simulink model "mainECU"  (R2015b)
settings: Solver=FixedStepDiscrete  StartTime=0.0  StopTime=Inf  FixedStep=0.001  RelTol=1e-3
PostLoadFcn:
  | , if any(exist('dsrtsu_mdlpostloadfcn', 'file') == [2, 3, 6]), try dsrtsu_mdlpostloadfcn('Execute', bdroot); catch fprintf('Error in PostLoadFcn (dsrtsu_mdlpostloadfcn) for model "%s":\n %s\n', bdroot, lasterr); end, end,
undefined symbols (not defined in the file or in its folder): STARTUP
libraries: dspswit3 x5, rtican x5, simulink x2
(part 1 of 2)
settings Model: DSRTSU_INTERNAL_RTI_VER=460  DSRTSU_INTERNAL_RTI_TYPE=rti1401  RTICANMMDATA=struct('GeneralSetupData',struct('modelroot','e:\working\ds1401\demos\model\ds1401\model','generalsettings',struct('filesettings',struct('destfolder',struct('Name','RTICANMM_FILES','Check',1),'buildfolder',struct('Name','.','Check',1),'AbsDestfolder',struct('Name','e:\working\ds1401\demos\model\ds1401\model\RTICANMM_FILES'),'AbsBuildfolder',struct('Name','e:\working\ds1401\demos\model\ds1401\model'))),'options',struct('addpaths',1,'rmpaths',1,'addtrcexclusion',logical(1),'cannavigator',struct('checkmonitoring',0),'show_usrtrc',0,'use_usrtrc',0),'advanced',struct('options',[1 1 1 1 1 1 1 1 1 1 1 1 1 1 1 1 1 1 1 1 1 1 1 1 1 1 1 1 1 1 1 1 1 1 1 1 1 1 1 1 1 1 1 1 1 1 1 1 1 1 1 1 1 1 1 1 1 1 1 1 1 1 1 1 1 1 1 1 1 1 1 1 1 1 1 1 1 1 1 1 1 1 1 1 1 1 1 1 1 1 1 1 1 1 1 1 1 1 1 1]),'MPSetup',{{}},'modelname','demo1401_throttle_control_1513','block','demo1401_throttle_control_1513'))  DSRTSU_INTERNAL_RTIFLEXRAYCONFIG=70  DSRTSU_INTERNAL_RTIFPGA=50  ExtModeTrigMode=oneshot  ExtModeArmWhenConnect=off  ExtModeAutoUpdateStatusClock=off  Creator=dSPACE GmbH  LastModifiedBy=luis
settings SolverCC: AutoInsertRateTranBlk=on
settings DataIOCC: SaveFormat=Array  SignalLoggingSaveFormat=ModelDataLogs
settings OptimizationCC: BlockReduction=off  ConditionallyExecuteInputs=off  OptimizeBlockIOStorage=off  BufferReuse=off  GlobalBufferReuse=off  ExpressionFolding=off  ExpressionDepthLimit=2147483647  LocalBlockOutputs=off  InitFltsAndDblsToZero=on
settings DebuggingCC: SaveWithParameterizedLinksMsg=none  UnderspecifiedInitializationDetection=Classic  MergeDetectMultiDrivingBlocksExec=none  SignalResolutionControl=TryResolveAllWithWarning  SolverPrmCheckMsg=warning  MultiTaskDSMMsg=warning  MultiTaskCondExecSysMsg=none  MultiTaskRateTransMsg=warning  TasksWithSamePriorityMsg=none  FcnCallInpInsideContextMsg=UseLocalSettings  StateNameClashWarn=warning
settings HardwareCC: ProdBitPerPointer=32  ProdLargestAtomicFloat=None  ProdEndianess=BigEndian  ProdWordSize=32  ProdHWDeviceType=Generic->Custom  TargetIntDivRoundTo=Zero  TargetEndianess=BigEndian  TargetHWDeviceType=Generic->Custom
settings RTWCC: SystemTargetFile=rti1401.tlc  MakeCommand=make_rti  TemplateMakefile=rti1401.tmf  Description=dSPACE DS1401 Hardware Platform  RTWVerbose=off
settings STFCustomTargetCC: ParMdlRefBuildCompliant=on  ConcurrentExecutionCompliant=off  GeneratePreprocessorConditionals=Use local settings  CPPClassGenCompliant=off  SystemTargetFile=rti1401.tlc
settings GRTTargetCC: CompOptLevelCompliant=off  ConcurrentExecutionCompliant=off  CombineOutputUpdateFcns=off  MatFileLogging=off  CPPClassGenCompliant=off  GRTInterface=on  UseToolchainInfoCompliant=off  ExtModeMexFile=noextcomm
settings ConfigComp: CovModelRefEnable=Off

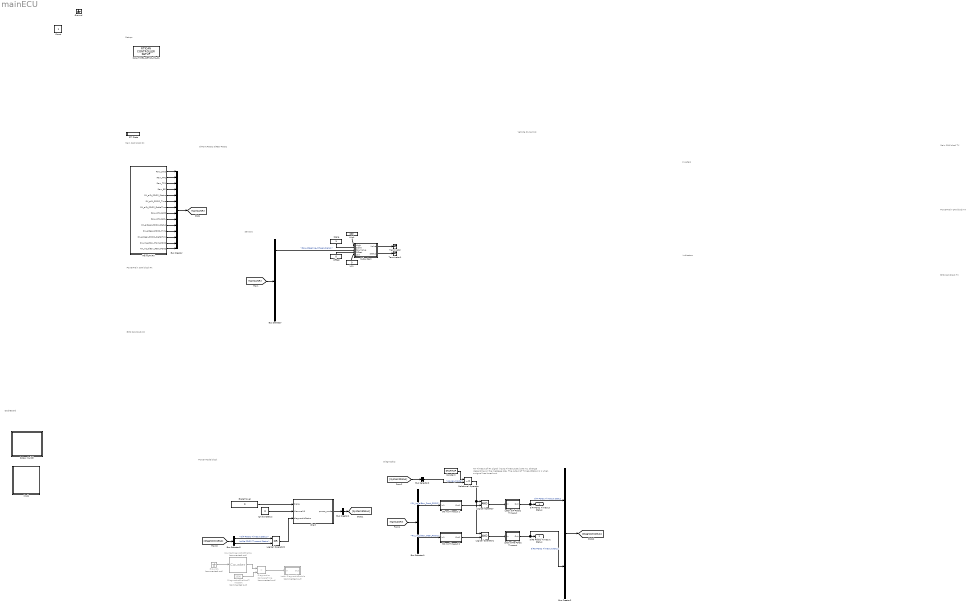
== system mainECU ==
  note: DashBoard
  note: Diagnostics
  note: RX Timeout of RX signal inputs
      | Timeout set is 50 ms. Change depending on the message rate.
      | The output of TimeoutStatus is 1 when a signal has timed out.
  note: aiFront PDO2
      | aiRear PDO2
  note: Sensors
  note: Power Mode block
  note: Main
      | CAN block
      | RX
  note: Setups
  note: PowerTrain
      | CAN block
      | RX
  note: BMS
      | CAN block
      | RX
  note: Vehicle Dynamics
  note: Indicators
  note: Inverters
  note: Main
      | CAN block
      | TX
  note: PowerTrain
      | CAN block
      | TX
  note: BMS
      | CAN block
      | TX
  50 ms Timeout 1 : Subsystem
  50 ms Timeout 2 : Subsystem
  BrakeTravel : Constant  Value=0
  Bus Creator : BusCreator  Inputs=14
  Bus Creator1 : BusCreator  Inputs=1
  Bus Creator2 : BusCreator  Inputs=2
  Bus Selector : BusSelector  OutputSignals=Raw_Steering_Wheel_Signal,Raw_Throttle_Pedal_2,Raw_Throttle_Pedal_1,Raw_Brake_Signal
  Bus Selector1 : BusSelector  OutputSignals=RX_Int_aiBox_Front_PDO2,RX_Int_aiBox_Rear_PDO2
  Bus Selector2 : BusSelector  OutputSignals=power_mode
  Bus Selector3 : BusSelector  OutputSignals=aiFr PDO2 Timeout Status,aiRe PDO2 Timeout Status
  CAN_TYPE1_SETUP_M1_C1 : rtican/RTICAN CONTROLLER SETUP   Reserved1=[]  Reserved2=[]  Reserved3=[]  Reserved4=[]  AcceptanceMask=[]  ArbitrationField=[]  Parameters=[]  SFcnRTICANSettings=[]  MS_Struct=[]  BoardTypeNo=[]  BoardNo=[]  ChannelNo=[]  DialogFcn=[]  UnitName=[]  Revision=[]  UnitValues=[]  DSProperties=struct('RTI',struct('Version',uint32(12),'BlockType',struct('isSLSource',uint8(0),'isSLSink',uint8(0),'isHWSource',uint8(0),'isHWSink',uint8(0),'isSetup',uint8(1),'isInline',uint8(1),'isNonInline',uint8(0),'isInterrupt',uint8(0),'isChannelwise',uint8(0)),'IOBoardType','RTICAN','UnitType','NON_MESSAGE','Identifier','MASTER','DialogType','ML','BlockSet','RTICAN','SlaveProcessor','CAN'))  RTIBlockInterface=struct('InputPortsWidth',int32(0),'InputPortsActive',0,'OutputPortsWidth',int32(0),'OutputPortsActive',0,'DialogFcn','rtican_master_setup_gui','BlockDisplay',{{['CAN CONTROLLER\n SETUP'],'center'}},'IconTransparency','on','InitLevel',3,'IWork',{{{'',uint32(2)}}},'BlockName',struct('Token',{{'CAN_TYPE','_SETUP_M','_C'}},'BlockParam',{{'BoardTypeNo','BoardNo','ChannelNo'}}),'ParameterTunableNames',{{}})  RTIBlockParameters="struct('BoardTypeNo',{{1,'OFF',[]}},'BoardNo',{{1,'ON',[1 16]}},'ChannelNo',{{1,'ON',[1 2]}},'AcceptanceMask',{{0,'OFF',[]}},'ArbitrationField',{{0,'OFF',[]}},'Parameters',{{struct('Config',struct('Baudrate',500,'SampleMode',1,'UsedParamSet',1,'validSettings',1,'isBTRvalues',0,'Advanced',struct('Baudrate',{500,500,500},'Frequency',{24000000,36000000,64000000},'Settings',{struct('SMPL',0,'BRP',0,'NBT',24,'TSEG1',15,'TSEG2',6,'SJW',3,'SP',70),struct('SMPL',0,'BRP',1,'NBT',18,'TSEG1',14,'TSEG2',1,'SJW',1,'SP',88),struct('SMPL',0,'BRP',3,'NBT',16,'TSEG1',12,'TSEG2',1,'SJW',1,'SP',87)},'BTR0',{192,65,67},'BTR1',{111,30,28})),'configType',1,'Options',struct('DataFileSelected',1,'DataFileName',{{'database\\main_0_2.dbc'}},'DataFileDate',{{['07-ene.-2017 20:06:27']}},'InterfaceFcn','rtican_dbc_file_parser','InterfaceFcnFileName','','LabelConfigType','volatile','AcceptanceMaskSelected',0,'MsgDataType','AllwaysDouble','NumType','hex','MaskType','STD','AcceptanceMask',0,'ArbitrationField',0,'UseMultipleMessageAccess',0),'RxReceiveStdOptions',struct('RxServiceStdEnabled',0,'RxServiceStdMsgIdent',1000,'RxServiceStdIdentNumType',1,'RxServiceStdIdentMask',0,'RxServiceStdMaskNumType',1,'RxServiceStdQueueSize',64),'RxReceiveXtdOptions',struct('RxServiceXtdEnabled',0,'RxServiceXtdMsgIdent',1001,'RxServiceXtdIdentNumType',1,'RxServiceXtdIdentMask',0,'RxServiceXtdMaskNumType',1,'RxServiceXtdQueueSize',64),'PartialNetworkingOptions',struct('switchedon',0,'format',1,'idmask',['    XXXXX XXXXXXXX XXXXXXXX XXXXXXXX'],'idcode','0','idfilter','0','datamaskused',0,'datalength',1,'datamask','0x0000000000000000','partialnetworkenable',0),'general',struct('Termination_common',1,'Termination_C252',1,'BusConfigurationRegister',0,'Transceiver','ISO11898','isFromLib',0)),'OFF',[]}},'CCPParameters',{{struct('CRO',struct('Format','STD','NumFormat','hex','Id',1639),'DTO',struct('Format','STD','NumFormat','hex','Id',2017),'StationAdr',struct('NumFormat','hex','Value',57),'StationId',struct('Value',['dSPACE CCP Service']),'Enabled',0),'OFF',[]}},'XCPParameters',{{struct('MASTER',struct('Format','STD','NumFormat','hex','Id',256),'SLAVE',struct('Format','STD','NumFormat','hex','Id',510),'Enabled',0,'PIDTransmissionEnabled',0),'OFF',[]}},'GroupId',{{struct('Group',{{'RTICAN'}},'No',1,'Behavior',{{'EVER'}},'BlockType',{{'SOURCE'}},'NameChangeFlag',1),'OFF',[]}},'SFcnRTICANSettings',{{struct('Baudrate',500,'configType',1,'AdvancedConfig',struct('Frequency',{},'BTR0',{},'BTR1',{}),'UsedParamSet',1,'STDMaskSelected','no','XTDMaskSelected','no','BoardType','DS1','BoardNo',1,'ControllerNo',1,'Transceiver','ISO11898','BusConfigRegister',0,'TerminationRes',120,'UseMultipleMessageAccess','no','STDRXSrvcUsed','no','STDRXSrvcMsgId',1000,'STDRXSrvcMsgMask',0,'STDRXSrvcQueueSize',64,'XTDRXSrvcUsed','no','XTDRXSrvcMsgId',1001,'XTDRXSrvcQueueSize',64,'XTDRXSrvcMsgMask',0,'PN_IsPNTransciever',0,'PN_IsPNEnabled',0,'PN_MsgFormat',1,'PN_idcode',0,'PN_idmask',2047,'PN_datamaskused',0,'PN_datalength',0,'PN_datamask',['0xFF, 0xFF, 0xFF, 0xFF, 0xFF, 0xFF, 0xFF, 0xFF']),'OFF',[]}},'SFcnRTICCPSettings',{{struct('CRO',struct('Format','STD','NumFormat','hex','Id',1639),'DTO',struct('Format','STD','NumFormat','hex','Id',2017),'StationAdr',struct('NumFormat','hex','Value',57),'StationId',struct('Value',['dSPACE CCP Service']),'Enabled',0),'OFF',[]}},'SFcnRTIXCPSettings',{{struct('MASTER',struct('Format','STD','NumFormat','hex','Id',256),'SLAVE',struct('Format','STD','NumFormat','hex','Id',510),'Enabled',0,'PIDTransmissionEnabled',0),'OFF',[]}},'TLCFileName',{{'rtican_master_setup','OFF',[]}})"  RTISFcnParameters=struct('SFcnRTICANSettings','struct','SFcnRTICCPSettings','struct','SFcnRTIXCPSettings','struct','AcceptanceMask','int32','ArbitrationField','int32','TLCFileName','char')  RTIBlockParaDefault="struct('BoardTypeNo',4302,'BoardNo',1,'ChannelNo',1,'AcceptanceMask',0,'ArbitrationField',0,'Parameters',struct('Config',struct('Baudrate',500,'SampleMode',1,'UsedParamSet',1,'validSettings',1,'isBTRvalues',0,'Advanced',struct('Frequency',16000000,'BTR0',64,'BTR1',28,'Settings',struct('SMPL',0,'BRP',0,'NBT',16,'TSEG1',12,'TSEG2',1,'SJW',1,'SP',87))),'configType',1,'Options',struct('DataFileSelected',0,'DataFileName',{{['<no datafile support>']}},'DataFileDate',{{''}},'InterfaceFcn','rtican_dbc_file_parser','InterfaceFcnFileName','','LabelConfigType','volatile','AcceptanceMaskSelected',0,'MsgDataType','AllwaysDouble','NumType','hex','MaskType','STD','AcceptanceMask',0,'ArbitrationField',0,'UseMultipleMessageAccess',0),'RxReceiveStdOptions',struct('RxServiceStdEnabled',0,'RxServiceStdMsgIdent',1000,'RxServiceStdIdentNumType',1,'RxServiceStdIdentMask',0,'RxServiceStdMaskNumType',1,'RxServiceStdQueueSize',64),'RxReceiveXtdOptions',struct('RxServiceXtdEnabled',0,'RxServiceXtdMsgIdent',1001,'RxServiceXtdIdentNumType',1,'RxServiceXtdIdentMask',0,'RxServiceXtdMaskNumType',1,'RxServiceXtdQueueSize',64),'PartialNetworkingOptions',struct('switchedon',0,'format',1,'idmask',['    XXXXX XXXXXXXX XXXXXXXX XXXXXXXX'],'idcode','0','idfilter','0','datamaskused',0,'datalength',1,'datamask','0x0000000000000000','partialnetworkenable',0),'general',struct('Termination_common',1,'Termination_C252',1,'BusConfigurationRegister',0,'Transceiver','ISO11898','isFromLib',1)),'CCPParameters',struct('CRO',struct('Format','STD','NumFormat','hex','Id',1639),'DTO',struct('Format','STD','NumFormat','hex','Id',2017),'StationAdr',struct('NumFormat','hex','Value',57),'StationId',struct('Value',['dSPACE CCP Service']),'Enabled',0),'XCPParameters',struct('MASTER',struct('Format','STD','NumFormat','hex','Id',256),'SLAVE',struct('Format','STD','NumFormat','hex','Id',510),'Enabled',0,'PIDTransmissionEnabled',0),'GroupId',struct('Group',{{'RTICAN'}},'No',1,'Behavior',{{'EVER'}},'BlockType',{{'SOURCE'}},'NameChangeFlag',1),'SFcnRTICANSettings',struct('Baudrate',500,'configType',1,'AdvandedConfig',struct('Frequency',16000000,'BTR0','0x40','BTR1','0x1C'),'UsedParamSet',1,'STDMaskSelected','no','XTDMaskSelected','no','BoardType','DS4302','BoardNo',1,'ControllerNo',1,'Transceiver','ISO11898','BusConfigRegister',0,'TerminationRes',120,'UseMultipleMessageAccess','no','STDRXSrvcUsed','no','STDRXSrvcMsgId',1000,'STDRXSrvcMsgMask',0,'STDRXSrvcQueueSize',64,'XTDRXSrvcUsed','no','XTDRXSrvcMsgId',1001,'XTDRXSrvcQueueSize',64,'XTDRXSrvcMsgMask',0),'SFcnRTICCPSettings',struct('CRO',struct('Format','STD','NumFormat','hex','Id',1639),'DTO',struct('Format','STD','NumFormat','hex','Id',2017),'StationAdr',struct('NumFormat','hex','Value',57),'StationId',struct('Value',['dSPACE CCP Service']),'Enabled',0),'SFcnRTIXCPSettings',struct('MASTER',struct('Format','STD','NumFormat','hex','Id',256),'SLAVE',struct('Format','STD','NumFormat','hex','Id',510),'Enabled',0,'PIDTransmissionEnabled',0),'TLCFileName','rtican_master_setup')"
      settings: AttributesFormatString=Group Id: RTICAN1\n
  Chart : Stateflow chart  TreatAsAtomicUnit=on
  Constant : Constant  Value=STARTUP
  CounterDiagnosticsEnable : dspswit3/Counter  Commented=on  Direction=Up  CountEvent=Free running  CounterSize=User defined  MaxCount=20000  InitialCount=0  Output=Count  HitValue=32  ResetInput=on  SamplesPerFrame=1  Ts=-1  CntDtype=double  HitDtype=Logical
  Diagnostics CompareTime : RelationalOperator  Commented=on  Operator=>  OutDataTypeStr=boolean
  DiagnosticsEnabledTimeStart : Constant  Commented=on  Value=2000
  Ground1 : Ground  Commented=on
  High : Constant  Value=100
  IgnitionStatus : Constant  Value=0
  Knob : Subsystem  DialogController=hmiCreateDDGDialog  IsWebBlock=on  mask(MWDashboardBlock){webBlockId=318b6eff-2907-45e0-b318-c643b2e3d79c, webBlockType=continuousknob, ShowInLibBrowser=on, ShowInitialText=on, HMISrcModelName=mainECU}
      mask prompts: webBlockId "WebBlock Id"; webBlockType "WebBlock Type"; HMISrcModelName "Source Model"
      mask Help: helpview([docroot '/mapfiles/simulink.map'], 'hmi_knob')
      mask Display:
      | if strcmp(get_param(bdroot(gcb),'BlockDiagramType'), 'library')
      |     image([(matlabroot) '/toolbox/simulink/hmi/icons/ContinuousKnob.png']);
      | end
  Latch DiagnosticEnable : Subsystem  Commented=on
  Latch aiFr PDO2 Timeout : Subsystem
  Latch aiRe PDO2 Timeout : Subsystem
  Logical Operator : Logic  AllPortsSameDT=off  OutDataTypeStr=boolean
  Logical Operator1 : Logic  AllPortsSameDT=off  OutDataTypeStr=boolean
  Logical Operator2 : Logic  Operator=OR  AllPortsSameDT=off  OutDataTypeStr=boolean
  Low : Constant  Value=0
  MainCAN RX : Subsystem
  Offset : Constant  Value=0
  RTI Data : Subsystem  Tag=struct('RTIDataServer',struct('RTIDataServerVs','2','RTIModelDescription','struct(''main'',''mainECU'',''sub'','''',''isMp'',0)'))  LoadFcn="if exist('rtidc'), try,  rtidc('DataHostBlockClbLoad', gcbh); catch, disp(['Warning: ''LoadFcn'' for RTI Data block failed: ' lasterr]); end, end,"  mask(RTI_DATA_HOST){}
      mask help:
      | RTI Data Block.
      | This block is used by RTI to store internal model-dependent data.
      | Please keep this block on the root level of the model. Deleting this block will result in data loss.
      |
      | NEVER DELETE OR COPY THIS BLOCK!
      settings: CopyFcn="if exist('rtidc'), try,  rtidc('DataHostBlockClbCopy', gcbh); catch, disp(['Warning: ''CopyFcn'' for RTI Data block failed: ' lasterr]); end, end,"  DeleteFcn="if exist('rtidc'), try,  rtidc('DataHostBlockClbDelete', gcbh); catch, disp(['Warning: ''DeleteFcn'' for RTI Data block failed: ' lasterr]); end, end,"  ModelCloseFcn="if exist('rtidc'), try,  rtidc('DataHostBlockClbModelClose', gcbh); catch, disp(['Warning: ''ModelCloseFcn'' for RTI Data block failed: ' lasterr]); end, end,"  PreSaveFcn="if exist('rtidc'), try,  rtidc('DataHostBlockClbPreSave', gcbh); catch, disp(['Warning: ''PreSaveFcn'' for RTI Data block failed: ' lasterr]); end, end,"  PostSaveFcn="if exist('rtidc'), try,  rtidc('DataHostBlockClbPostSave', gcbh); catch, disp(['Warning: ''PostSaveFcn'' for RTI Data block failed: ' lasterr]); end, end,"  NameChangeFcn="if exist('rtidc'), try,  rtidc('DataHostBlockClbNameChange', gcbh); catch, disp(['Warning: ''NameChangeFcn'' for RTI Data block failed: ' lasterr]); end, end,"
      mask Help:
      | RTI Data Block.
      | This block is used by RTI to store internal model-dependent data.
      | Please keep this block on the root level of the model. Deleting this block will result in data loss.
      | 
      | NEVER DELETE OR COPY THIS BLOCK!
      mask Display:
      | text(0.5, 0.5, 'RTI Data', 'HorizontalAlignment', 'center');
      | plot([1 0]);
  Relational Operator : RelationalOperator  Operator=~=  OutDataTypeStr=boolean
  Rotary Switch : Subsystem  DialogController=hmiCreateDDGDialog  IsWebBlock=on  mask(MWDashboardBlock){webBlockId=394b7d7a-f303-4d15-a706-6c693a0bf5c3, webBlockType=discreteknob, ShowInLibBrowser=on, ShowInitialText=on, HMISrcModelName=mainECU}
      mask prompts: webBlockId "WebBlock Id"; webBlockType "WebBlock Type"; HMISrcModelName "Source Model"
      mask Help: helpview([docroot '/mapfiles/simulink.map'], 'hmi_rotary_switch')
      mask Display:
      | model = bdroot(gcb);
      | if strcmp(get_param(model,'BlockDiagramType'), 'library')
      |     image([(matlabroot) '/toolbox/simulink/hmi/icons/DiscreteKnob.png']);
      | end
  Scale : Constant
  Subsystem : Subsystem
  Terminator : Terminator
  Terminator1 : Terminator
  aiFr PDO2 Timeout Status : Outport
  aiRe PDO2 Timeout Status : Outport  Port=2
  Const : Constant  IOType=siggen
  Ground : Ground  IOType=siggen
  tag scope: MainCANRX=global
  wires:
  MainCAN RX/6(RX_aiFr_PDO2_Time) -> Bus Creator/6
  MainCAN RX/1(Raw_SWS) -> Bus Creator/1
  MainCAN RX/2(Raw_TP2) -> Bus Creator/2
  MainCAN RX/3(Raw_TP1) -> Bus Creator/3
  MainCAN RX/4("Raw_BS ") -> Bus Creator/4
  MainCAN RX/5(RX_aiFr_PDO2_Status) -> Bus Creator/5
  MainCAN RX/7(RX_aiFr_PDO2_DeltaTime) -> Bus Creator/7
  MainCAN RX/8(Raw_WSuspRR) -> Bus Creator/8
  MainCAN RX/9(Raw_WSuspRL) -> Bus Creator/9
  MainCAN RX/10(RX_aiRear_PDO2_Status) -> Bus Creator/10
  MainCAN RX/11(RX_aiRear_PDO2_Time) -> Bus Creator/11
  MainCAN RX/12(RX_aiRear_PDO2_DeltaTime) -> Bus Creator/12
  [MainCANRX] -> Bus Selector/1
  Bus Creator/1 -> [MainCANRX]
  [MainCANRX] -> Bus Selector1/1
  MainCAN RX/13(RX_Int_aiBox_Front_PDO2) -> Bus Creator/13
  MainCAN RX/14(RX_Int_aiBox_Rear_PDO2) -> Bus Creator/14
  Bus Selector1/2 -> 50 ms Timeout 2/1(In1)  "<RX_Int_aiBox_Rear_PDO2>"
  Bus Selector1/1 -> 50 ms Timeout 1/1(In1)  "<RX_Int_aiBox_Front_PDO2>"
  50 ms Timeout 1/1(Out1) -> Logical Operator/2
  [SystemStatus] -> Bus Selector2/1
  Bus Creator1/1 -> [SystemStatus]
  50 ms Timeout 2/1(Out1) -> Logical Operator1/2
  Ground1/1 -> CounterDiagnosticsEnable/1
  DiagnosticsEnabledTimeStart/1 -> Diagnostics CompareTime/2
  CounterDiagnosticsEnable/1 -> Diagnostics CompareTime/1
  Logical Operator1/1 -> Latch aiRe PDO2 Timeout/1(In)
  Logical Operator/1 -> Latch aiFr PDO2 Timeout/1(In)
  Latch aiFr PDO2 Timeout/1(Out) -> Bus Creator2/1, aiFr PDO2 Timeout Status/1  "aiFr PDO2 Timeout Status"
  Latch aiRe PDO2 Timeout/1(Out) -> Bus Creator2/2, aiRe PDO2 Timeout Status/1  "aiRe PDO2 Timeout Status"
  Diagnostics CompareTime/1 -> Latch DiagnosticEnable/1(In)
  High/1 -> Subsystem/1(High)
  Scale/1 -> Subsystem/2(Scale)
  Bus Selector/1 -> Subsystem/3(RawValue)  "<Raw_Steering_Wheel_Signal>"
  Offset/1 -> Subsystem/4(Offset)
  Low/1 -> Subsystem/5(Low)
  Subsystem/1(Value) -> Terminator/1
  Subsystem/2(Status) -> Terminator1/1
  Chart/1(power_mode) -> Bus Creator1/1
  IgnitionStatus/1 -> Chart/2(klemme15)
  BrakeTravel/1 -> Chart/1(brake)
  Bus Creator2/1 -> [DiagnosticsBus]
  [DiagnosticsBus] -> Bus Selector3/1
  Bus Selector3/1 -> Logical Operator2/1  "<aiFr PDO2 Timeout Status>"
  Bus Selector3/2 -> Logical Operator2/2  "<aiRe PDO2 Timeout Status>"
  Logical Operator2/1 -> Chart/3(diagnosticStatus)
  Relational Operator/1 -> Logical Operator1/1, Logical Operator/1
  Bus Selector2/1 -> Relational Operator/2  "<power_mode>"
  Constant/1 -> Relational Operator/1

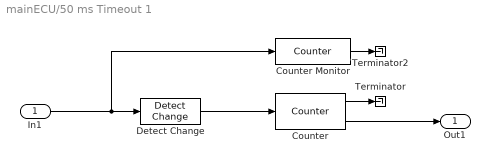
== system mainECU/50 ms Timeout 1 ==
  In1 : Inport
  Counter : dspswit3/Counter  Direction=Up  CountEvent=Free running  CounterSize=User defined  MaxCount=65535  InitialCount=0  Output=Count and Hit  HitValue=55  ResetInput=on  SamplesPerFrame=1  Ts=-1  CntDtype=double  HitDtype=Boolean
  Counter Monitor : dspswit3/Counter  Direction=Up  CountEvent=Either edge  CounterSize=User defined  MaxCount=100000  InitialCount=0  Output=Count  HitValue=32  ResetInput=off  SamplesPerFrame=1  Ts=1  CntDtype=double  HitDtype=Logical
  Detect Change : simulink/Logic and Bit Operations/Detect Change  vinit=0  InputProcessing=Inherited  OutDataTypeStr=uint8
  Terminator : Terminator
  Terminator2 : Terminator
  Out1 : Outport
  wires:
  Counter Monitor/1 -> Terminator2/1
  Counter/2 -> Out1/1
  Counter/1 -> Terminator/1
  In1/1 -> Counter Monitor/1, Detect Change/1
  Detect Change/1 -> Counter/1

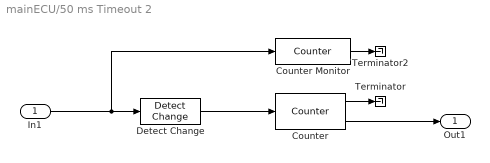
== system mainECU/50 ms Timeout 2 ==
  In1 : Inport
  Counter : dspswit3/Counter  Direction=Up  CountEvent=Free running  CounterSize=User defined  MaxCount=65535  InitialCount=0  Output=Count and Hit  HitValue=55  ResetInput=on  SamplesPerFrame=1  Ts=-1  CntDtype=double  HitDtype=Boolean
  Counter Monitor : dspswit3/Counter  Direction=Up  CountEvent=Either edge  CounterSize=User defined  MaxCount=100000  InitialCount=0  Output=Count  HitValue=32  ResetInput=off  SamplesPerFrame=1  Ts=1  CntDtype=double  HitDtype=Logical
  Detect Change : simulink/Logic and Bit Operations/Detect Change  vinit=0  InputProcessing=Inherited  OutDataTypeStr=uint8
  Terminator : Terminator
  Terminator2 : Terminator
  Out1 : Outport
  wires:
  Counter Monitor/1 -> Terminator2/1
  Counter/2 -> Out1/1
  Counter/1 -> Terminator/1
  In1/1 -> Counter Monitor/1, Detect Change/1
  Detect Change/1 -> Counter/1

== system mainECU/Knob ==

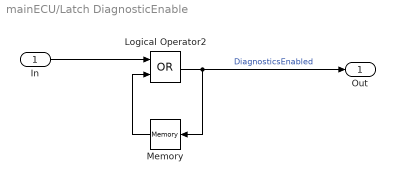
== system mainECU/Latch DiagnosticEnable ==
  In : Inport  OutDataTypeStr=boolean
  Logical Operator2 : Logic  Operator=OR  OutDataTypeStr=boolean
  Memory : Memory  X0=false
  Out : Outport
  wires:
  Memory/1 -> Logical Operator2/2
  Logical Operator2/1 -> Out/1, Memory/1  "DiagnosticsEnabled"
  In/1 -> Logical Operator2/1

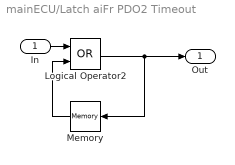
== system mainECU/Latch aiFr PDO2 Timeout ==
  In : Inport
  Logical Operator2 : Logic  Operator=OR  AllPortsSameDT=off  OutDataTypeStr=boolean
  Memory : Memory
  Out : Outport
  wires:
  Memory/1 -> Logical Operator2/2
  In/1 -> Logical Operator2/1
  Logical Operator2/1 -> Memory/1, Out/1

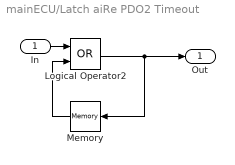
== system mainECU/Latch aiRe PDO2 Timeout ==
  In : Inport
  Logical Operator2 : Logic  Operator=OR  AllPortsSameDT=off  OutDataTypeStr=boolean
  Memory : Memory
  Out : Outport
  wires:
  Memory/1 -> Logical Operator2/2
  In/1 -> Logical Operator2/1
  Logical Operator2/1 -> Memory/1, Out/1

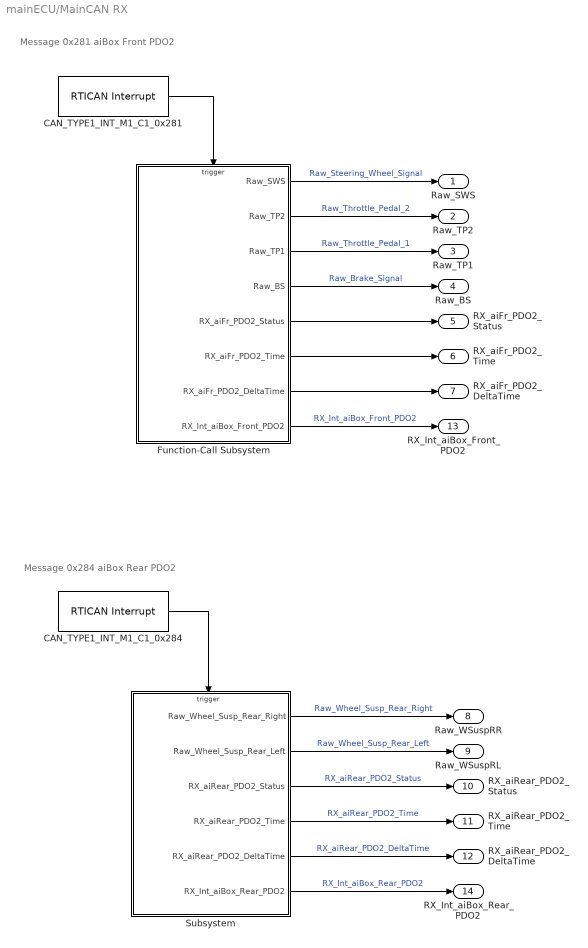
== system mainECU/MainCAN RX ==
  note: Message 0x284 aiBox Rear PDO2
  note: Message 0x281 aiBox Front PDO2
  CAN_TYPE1_INT_M1_C1_0x281 : rtican/RTICAN Interrupt  Reserved1=[]  Reserved2=[]  Reserved3=[]  Reserved4=[]  BoardTypeNo=[]  BoardNo=[]  ChannelNo=[]  Parameters=[]  InterruptName=[]  BoardIntNo=[]  Sfcn_Int_Struct=[]  BoardType=[]  SintNo=[]  Int_Struct=[]  DialogFcn=[]  UnitName=[]  Revision=[]  UnitValues=[]  DSProperties=struct('RTI',struct('Version',uint32(4),'BlockType',struct('isSLSource',uint8(1),'isSLSink',uint8(0),'isHWSource',uint8(1),'isHWSink',uint8(0),'isSetup',uint8(0),'isInline',uint8(1),'isNonInline',uint8(0),'isInterrupt',uint8(1),'isChannelwise',uint8(0)),'IOBoardType','RTICAN','UnitType','HWINT','Identifier','CANINT','DialogType','ML','BlockSet','RTICAN','RelationId',struct('TH',struct('BlockId','HWINT')),'SlaveProcessor','CAN'))  RTIBlockInterface=struct('OutputPortsWidth',int32(1),'FunctionCall',uint32(0),'OutputPortsActive',1,'DialogFcn','rtican_interrupt_gui','BlockDisplay',{{['CAN RX Interrupt'],'center'}},'IconTransparency','off','ParameterTunableNames',{{}},'InitLevel',3,'BlockName',struct('Token',{{'CAN_TYPE','_INT_M','_C'}},'BlockParam',{{'BoardTypeNo','BoardNo','ChannelNo'}}),'Options',{{'SS_OPTION_FORCE_NONINLINED_FCNCALL','SS_OPTION_ASYNCHRONOUS_INTERRUPT'}})  RTIBlockParameters=struct('BoardTypeNo',{{1,'OFF',[]}},'BoardNo',{{1,'ON',[1 16]}},'ChannelNo',{{1,'ON',[1 2]}},'Parameters',{{struct('general',struct('Type','RX','NumFormat','hex','MsgIdFormat','STD','MsgId',641,'isFromLib',0)),'OFF',[]}},'GroupId',{{struct('Group','RTICAN','No',1,'Behavior','NAMECHANGE','BlockType','SINK','NameChangeFlag',0),'OFF',[]}},'SFcnRTICANInterrupt',{{0,'OFF',[]}},'ThSrcSgnName',{{['CAN_TYPE1_M1_C1 RX Interrupt'],'OFF',[]}},'ThBlk',{{['struct(''blkh'',[''mainECU/MainCAN RX/CAN_TYPE1_INT_M1_C1_0x281''],''srcId'',''CAN1'',''srcSgnId'',''CAN1'',''intervalTmrBlockId'',[],''srcSgnName'',[''CAN_TYPE1_M1_C1 RX Interrupt''],''srcCpuId'','''',''isSrcCpu'',1,''isTargetCpu'',1,''srcOnMasterCpu'',1,''boardType'',''CAN'',''boardTypeNo'',''1'',''boardNo'',0,''intNo'',0,''subIntNo'',-1,''period'',0,''entryPoint'',''rti_CAN1'',''blockName'',''CAN_TYPE1_INT_M1_C1_0x281'',''taskNameDisplayExt'','''',''taskType'',''HWINT'',''groupId'',''CANINT1B1'',''hookFcn'',''NULL'',''isTimerTaskSrc'',0,''service'','''',''mpBlkId'','''',''taskPriorityPreConfig'',''none'',''taskPriority'',-1,''taskSortWeighting'',[],''taskSchedulingPolicy'',''FCFS'',''taskOvrPreConfig'',''none'',''taskOvrStrategy'',1,''taskOvrQueueSize'',1,''taskVisibility'',''on'',''taskGroupId'','''',''taskGroupDisplayOrder'',[],''serviceDynamicGen'',0,''disableCodeGen'',0,''boardBase'',''0'',''noBoardBase'','''')'],'OFF',[]}},'PHSBoardBaseId',{{'DS4302','OFF',[]}},'TLCFileName',{{'rtican_interrupt','OFF',[]}})  RTISFcnParameters=struct('SFcnRTICANInterrupt','struct','ThBlk','struct','PHSBoardBaseId','char','TLCFileName','char')  RTIBlockParaDefault=struct('BoardTypeNo',4302,'BoardNo',1,'ChannelNo',1,'Parameters',struct('general',struct('Type','RX','NumFormat','dec','MsgIdFormat','STD','MsgId',100,'isFromLib',1)),'GroupId',struct('Group',{{'RTICAN'}},'No',1,'Behavior',{{'NAMECHANGE'}},'BlockType',{{'SINK'}},'NameChangeFlag',0),'SFcnRTICANInterrupt',0,'ThSrcSgnName',['DS4302CAN_B1_C1 RX Interrupt'],'ThBlk',['struct(''srcSgnId'', '''')'],'PHSBoardBaseId','DS4302','TLCFileName','rtican_interrupt')
      settings: AttributesFormatString=Group Id: RTICAN1\n
  CAN_TYPE1_INT_M1_C1_0x284 : rtican/RTICAN Interrupt  Reserved1=[]  Reserved2=[]  Reserved3=[]  Reserved4=[]  BoardTypeNo=[]  BoardNo=[]  ChannelNo=[]  Parameters=[]  InterruptName=[]  BoardIntNo=[]  Sfcn_Int_Struct=[]  BoardType=[]  SintNo=[]  Int_Struct=[]  DialogFcn=[]  UnitName=[]  Revision=[]  UnitValues=[]  DSProperties=struct('RTI',struct('Version',uint32(4),'BlockType',struct('isSLSource',uint8(1),'isSLSink',uint8(0),'isHWSource',uint8(1),'isHWSink',uint8(0),'isSetup',uint8(0),'isInline',uint8(1),'isNonInline',uint8(0),'isInterrupt',uint8(1),'isChannelwise',uint8(0)),'IOBoardType','RTICAN','UnitType','HWINT','Identifier','CANINT','DialogType','ML','BlockSet','RTICAN','RelationId',struct('TH',struct('BlockId','HWINT')),'SlaveProcessor','CAN'))  RTIBlockInterface=struct('OutputPortsWidth',int32(1),'FunctionCall',uint32(0),'OutputPortsActive',1,'DialogFcn','rtican_interrupt_gui','BlockDisplay',{{['CAN RX Interrupt'],'center'}},'IconTransparency','off','ParameterTunableNames',{{}},'InitLevel',3,'BlockName',struct('Token',{{'CAN_TYPE','_INT_M','_C'}},'BlockParam',{{'BoardTypeNo','BoardNo','ChannelNo'}}),'Options',{{'SS_OPTION_FORCE_NONINLINED_FCNCALL','SS_OPTION_ASYNCHRONOUS_INTERRUPT'}})  RTIBlockParameters=struct('BoardTypeNo',{{1,'OFF',[]}},'BoardNo',{{1,'ON',[1 16]}},'ChannelNo',{{1,'ON',[1 2]}},'Parameters',{{struct('general',struct('Type','RX','NumFormat','hex','MsgIdFormat','STD','MsgId',644,'isFromLib',0)),'OFF',[]}},'GroupId',{{struct('Group','RTICAN','No',1,'Behavior','NAMECHANGE','BlockType','SINK','NameChangeFlag',0),'OFF',[]}},'SFcnRTICANInterrupt',{{0,'OFF',[]}},'ThSrcSgnName',{{['CAN_TYPE1_M1_C1 RX Interrupt'],'OFF',[]}},'ThBlk',{{['struct(''blkh'',[''mainECU/MainCAN RX/CAN_TYPE1_INT_M1_C1_0x284''],''srcId'',''CAN2'',''srcSgnId'',''CAN2'',''intervalTmrBlockId'',[],''srcSgnName'',[''CAN_TYPE1_M1_C1 RX Interrupt''],''srcCpuId'','''',''isSrcCpu'',1,''isTargetCpu'',1,''srcOnMasterCpu'',1,''boardType'',''CAN'',''boardTypeNo'',''1'',''boardNo'',0,''intNo'',1,''subIntNo'',-1,''period'',0,''entryPoint'',''rti_CAN2'',''blockName'',''CAN_TYPE1_INT_M1_C1_0x284'',''taskNameDisplayExt'','''',''taskType'',''HWINT'',''groupId'',''CANINT1B1'',''hookFcn'',''NULL'',''isTimerTaskSrc'',0,''service'','''',''mpBlkId'','''',''taskPriorityPreConfig'',''none'',''taskPriority'',-1,''taskSortWeighting'',[],''taskSchedulingPolicy'',''FCFS'',''taskOvrPreConfig'',''none'',''taskOvrStrategy'',1,''taskOvrQueueSize'',1,''taskVisibility'',''on'',''taskGroupId'','''',''taskGroupDisplayOrder'',[],''serviceDynamicGen'',0,''disableCodeGen'',0,''boardBase'',''0'',''noBoardBase'','''')'],'OFF',[]}},'PHSBoardBaseId',{{'DS4302','OFF',[]}},'TLCFileName',{{'rtican_interrupt','OFF',[]}})  RTISFcnParameters=struct('SFcnRTICANInterrupt','struct','ThBlk','struct','PHSBoardBaseId','char','TLCFileName','char')  RTIBlockParaDefault=struct('BoardTypeNo',4302,'BoardNo',1,'ChannelNo',1,'Parameters',struct('general',struct('Type','RX','NumFormat','dec','MsgIdFormat','STD','MsgId',100,'isFromLib',1)),'GroupId',struct('Group',{{'RTICAN'}},'No',1,'Behavior',{{'NAMECHANGE'}},'BlockType',{{'SINK'}},'NameChangeFlag',0),'SFcnRTICANInterrupt',0,'ThSrcSgnName',['DS4302CAN_B1_C1 RX Interrupt'],'ThBlk',['struct(''srcSgnId'', '''')'],'PHSBoardBaseId','DS4302','TLCFileName','rtican_interrupt')
      settings: AttributesFormatString=Group Id: RTICAN1\n
  Function-Call Subsystem : Subsystem  TreatAsAtomicUnit=on
  Subsystem : Subsystem
  Raw_SWS : Outport
  Raw_TP2 : Outport  Port=2
  Raw_TP1 : Outport  Port=3
  "Raw_BS " : Outport  Port=4
  RX_aiFr_PDO2_Status : Outport  Port=5
  RX_aiFr_PDO2_Time : Outport  Port=6
  RX_aiFr_PDO2_DeltaTime : Outport  Port=7
  Raw_WSuspRR : Outport  Port=8
  Raw_WSuspRL : Outport  Port=9
  RX_aiRear_PDO2_Status : Outport  Port=10
  RX_aiRear_PDO2_Time : Outport  Port=11
  RX_aiRear_PDO2_DeltaTime : Outport  Port=12
  RX_Int_aiBox_Front_PDO2 : Outport  Port=13
  RX_Int_aiBox_Rear_PDO2 : Outport  Port=14
  wires:
  Function-Call Subsystem/5(RX_aiFr_PDO2_Status) -> RX_aiFr_PDO2_Status/1
  Function-Call Subsystem/6(RX_aiFr_PDO2_Time) -> RX_aiFr_PDO2_Time/1
  Function-Call Subsystem/7(RX_aiFr_PDO2_DeltaTime) -> RX_aiFr_PDO2_DeltaTime/1
  Function-Call Subsystem/2(Raw_TP2) -> Raw_TP2/1  "Raw_Throttle_Pedal_2"
  Function-Call Subsystem/3(Raw_TP1) -> Raw_TP1/1  "Raw_Throttle_Pedal_1"
  Function-Call Subsystem/1(Raw_SWS) -> Raw_SWS/1  "Raw_Steering_Wheel_Signal"
  Function-Call Subsystem/4("Raw_BS ") -> "Raw_BS "/1  "Raw_Brake_Signal"
  CAN_TYPE1_INT_M1_C1_0x281/1 -> Function-Call Subsystem/Trigger
  Function-Call Subsystem/8(RX_Int_aiBox_Front_PDO2) -> RX_Int_aiBox_Front_PDO2/1  "RX_Int_aiBox_Front_PDO2"
  Subsystem/6(RX_Int_aiBox_Rear_PDO2) -> RX_Int_aiBox_Rear_PDO2/1  "RX_Int_aiBox_Rear_PDO2"
  CAN_TYPE1_INT_M1_C1_0x284/1 -> Subsystem/Trigger
  Subsystem/1(Raw_Wheel_Susp_Rear_Right) -> Raw_WSuspRR/1  "Raw_Wheel_Susp_Rear_Right"
  Subsystem/2(Raw_Wheel_Susp_Rear_Left) -> Raw_WSuspRL/1  "Raw_Wheel_Susp_Rear_Left"
  Subsystem/3(RX_aiRear_PDO2_Status) -> RX_aiRear_PDO2_Status/1  "RX_aiRear_PDO2_Status"
  Subsystem/4(RX_aiRear_PDO2_Time) -> RX_aiRear_PDO2_Time/1  "RX_aiRear_PDO2_Time"
  Subsystem/5(RX_aiRear_PDO2_DeltaTime) -> RX_aiRear_PDO2_DeltaTime/1  "RX_aiRear_PDO2_DeltaTime"

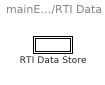
== system mainECU/RTI Data ==
  RTI Data Store : Subsystem  Tag="struct('private',struct('version',struct('dsVer',uint32(2),'dsVerCreation',uint32(2),'RTI',struct('ver','3.6.0b5','type','RTI1401')),'access',struct('type','Model','isPerm',1,'created',['29-Sep-2000 10:18:57'],'modified',['23-Jan-2017 15:09:16'],'location','')),'public',struct('main',struct('data',[]),'sub',struct('name',{{'mainECU'}},'data',{{struct('TH',struct('thTaskInfo',struct('taskType',{'TIMER','HWINT','TMRINT','SWINT','GLINT'},'tasksNumOf',{1,2,0,0,0},'srcIds',{{'TIMERA'},{'CAN1','CAN2'},{},{},{}},'taskNames',{{['Timer Task 1']},{'CAN_TYPE1_INT_M1_C1_0x281','CAN_TYPE1_INT_M1_C1_0x284'},{},{},{}})),'th_tc',struct('dataType',{'TASK','TASK','TASK'},'taskGroupId',{'','',''},'taskGroupList',{{},{},{}},'taskSchedulingPolicy',{'FCFS','FCFS','FCFS'},'taskType',{'TIMER','HWINT','HWINT'},'blkh',{-1,['mainECU/MainCAN RX/CAN_TYPE1_INT_M1_C1_0x281'],['mainECU/MainCAN RX/CAN_TYPE1_INT_M1_C1_0x284']},'srcId',{'TIMERA','CAN1','CAN2'},'srcSgnName',{['Timer A interrupt'],['CAN_TYPE1_M1_C1 RX Interrupt'],['CAN_TYPE1_M1_C1 RX Interrupt']},'srcCpuName',{'','',''},'taskName',{['Timer Task 1  [0.001] s'],'CAN_TYPE1_INT_M1_C1_0x281','CAN_TYPE1_INT_M1_C1_0x284'},'taskNameDisplayExt',{'','',''},'smplTime',{0.001,0,0},'smplTimeOffs',{0,0,0},'hasFixedPriority',{0,0,0},'priority',{1,2,3},'hasFixedOvc',{0,0,0},'ovcType',{1,1,1},'ovcMax',{0,1,1}),'tc_th',struct('dataType',{'TASK','TASK','TASK'},'taskGroupId',{'','',''},'taskGroupList',{{},{},{}},'taskSchedulingPolicy',{'FCFS','FCFS','FCFS'},'taskType',{'TIMER','HWINT','HWINT'},'blkh',{-1,['mainECU/MainCAN RX/CAN_TYPE1_INT_M1_C1_0x281'],['mainECU/MainCAN RX/CAN_TYPE1_INT_M1_C1_0x284']},'srcId',{'TIMERA','CAN1','CAN2'},'srcSgnName',{['Timer A interrupt'],['CAN_TYPE1_M1_C1 RX Interrupt'],['CAN_TYPE1_M1_C1 RX Interrupt']},'srcCpuName',{'','',''},'taskName',{['Timer Task 1  [0.001] s'],'CAN_TYPE1_INT_M1_C1_0x281','CAN_TYPE1_INT_M1_C1_0x284'},'taskNameDisplayExt',{'','',''},'smplTime',{0.001,0,0},'smplTimeOffs',{0,0,0},'hasFixedPriority',{0,0,0},'priority',{1,2,3},'hasFixedOvc',{0,0,0},'ovcType',{1,1,1},'ovcMax',{0,1,1}))}})))"  mask(RTI_DATA_STORE){}
      mask help:
      | RTI Data Store Block. This block is used by RTI to store internal model dependent data. Deleting this block will result in data loss.
      |
      | NEVER DELETE, COPY, OR MODIFY THIS BLOCK!
      mask Help:
      | RTI Data Store Block. This block is used by RTI to store internal model dependent data. Deleting this block will result in data loss.
      | 
      | NEVER DELETE, COPY, OR MODIFY THIS BLOCK!
      mask Display: text(0.5, 0.5, ' ', 'HorizontalAlignment', 'center');

== system mainECU/Rotary Switch ==

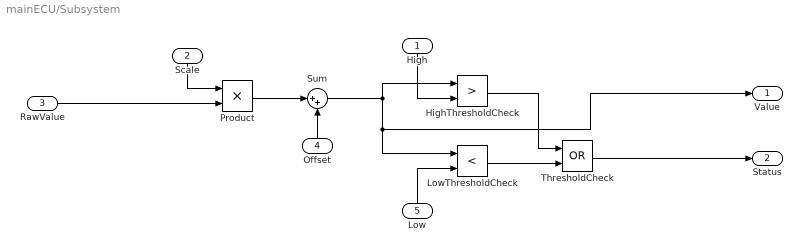
== system mainECU/Subsystem ==
  High : Inport
  Scale : Inport  Port=2
  RawValue : Inport  Port=3
  Offset : Inport  Port=4
  Low : Inport  Port=5
  HighThresholdCheck : RelationalOperator  Operator=>  OutDataTypeStr=boolean
  LowThresholdCheck : RelationalOperator  Operator=<  OutDataTypeStr=boolean
  Product : Product
  Sum : Sum  Inputs=|++
  ThresholdCheck : Logic  Operator=OR  AllPortsSameDT=off  OutDataTypeStr=boolean
  Value : Outport
  Status : Outport  Port=2
  wires:
  HighThresholdCheck/1 -> ThresholdCheck/1
  Offset/1 -> Sum/2
  ThresholdCheck/1 -> Status/1
  High/1 -> HighThresholdCheck/2
  Sum/1 -> Value/1, LowThresholdCheck/1, HighThresholdCheck/1
  Scale/1 -> Product/1
  Product/1 -> Sum/1
  Low/1 -> LowThresholdCheck/2
  RawValue/1 -> Product/2
  LowThresholdCheck/1 -> ThresholdCheck/2

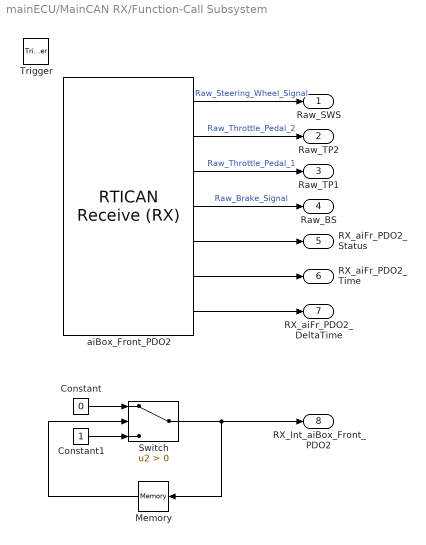
== system mainECU/MainCAN RX/Function-Call Subsystem ==
  Trigger : TriggerPort  TriggerType=function-call  OutputDataType=double
  Constant : Constant  Value=0
  Constant1 : Constant
  Memory : Memory  InheritSampleTime=on
  Switch : Switch  Criteria=u2 > Threshold
  aiBox_Front_PDO2 : rtican/RTICAN Receive (RX)   Reserved1=[]  Reserved2=[]  Reserved3=[]  Reserved4=[]  SfcnMessage=[]  Msg_Struct=[]  BoardTypeNo=[]  BoardNo=[]  ChannelNo=[]  Parameters=[]  DialogFcn=[]  UnitName=[]  Revision=[]  UnitValues=[]  DSProperties=struct('RTI',struct('Version',uint32(5),'BlockType',struct('isSLSource',uint8(1),'isSLSink',uint8(1),'isHWSource',uint8(0),'isHWSink',uint8(0),'isSetup',uint8(0),'isInline',uint8(1),'isNonInline',uint8(0),'isInterrupt',uint8(0),'isChannelwise',uint8(0)),'IOBoardType','RTICAN','UnitType','MESSAGE','Identifier','RX','DialogType','MSVC','BlockSet','RTICAN','SlaveProcessor','CAN'))  RTIBlockInterface=struct('OutputPortsWidth',int32([1 1 1 1 1 1 1]),'OutputPortsActive',[1 1 1 1 1 1 1],'OutputPortsName',{{'Raw_Steering_Wheel_Signal','Raw_Throttle_Pedal_2','Raw_Throttle_Pedal_1','Raw_Brake_Signal',['RX status'],['RX time'],['RX delta time']}},'OutputPortsDataType',{{'SS_DOUBLE','SS_DOUBLE','SS_DOUBLE','SS_DOUBLE','SS_DOUBLE','SS_DOUBLE','SS_DOUBLE'}},'OutputPortsLabel',{{'Raw_Steering_Wheel_Signal','Raw_Throttle_Pedal_2','Raw_Throttle_Pedal_1','Raw_Brake_Signal','','',''}},'OutputPortsLabelMode','ON','InputPortsWidth',int32(0),'InputPortsActive',0,'DialogFcn','rtican_message_interface_gui','BlockDisplay',{{'','center'}},'IconTransparency','on','ParameterTunableNames',{{}},'InitLevel',3,'BlockName',struct('Token',{{'aiBox_Front_PDO2'}}),'SampleTime',{{-1}},'TriggerPort',{{'none'}},'EnablePort',{{'none'}})  RTIBlockParameters=struct('BoardTypeNo',{{1,'OFF',[]}},'BoardNo',{{1,'ON',[1 16]}},'ChannelNo',{{1,'ON',[1 2]}},'Parameters',{{struct('DataFileSupport',struct('DataFileSelectedMaster',1,'DataFileSelectedLocal',1,'DataFileName',['c:\users\luis\documents\tuc racing\mainecu\database\main_0_2.dbc|'],'DataFileDate',{{{['07-ene.-2017 20:06:27']}}},'SelectedFile','database\main_0_2.dbc'),'Options',struct('StatusSelected',1,'TimeSelected',1,'DeltaTimeSelected',1,'BytePortSelected',0,'MessageLengthSelected',0,'TriggerPort',struct('Selected',0,'TriggerType',0),'UserCoding',struct('Selected',0,'InterfaceFile','UserDecodingFile','FcnName','UserDecodeFcn','InportSelected',0,'InportWidth',1,'OutportSelected',0,'OutportWidth',1),'EnablePortSelected',0,'SignalOnPortnameSelected',1,'UseRXService',0),'Message',struct('MsgOnBlocknameSelected',1,'MsgName','aiBox_Front_PDO2','MsgIdFormat',0,'MsgId',641,'MsgLength',8,'NumSignals',4,'SampleTime',-1,'Signal',struct('SgnName',{'Raw_Steering_Wheel_Signal','Raw_Throttle_Pedal_2','Raw_Throttle_Pedal_1','Raw_Brake_Signal'},'SgnStartBit',{0,16,32,48},'SgnLength',{16,16,16,16},'SgnType',{0,0,0,0},'ModeValue',{-1,-1,-1,-1},'DataType',{0,0,0,0},'ByteLayout',{2,2,2,2},'Factor',{1,1,1,1},'Offset',{0,0,0,0},'SgnComment',{{''},{''},{''},{''}},'SgnUnit',{'','','',''},'Min',{0,0,0,0},'Max',{0,0,0,0},'SLDataType',{'SS_DOUBLE','SS_DOUBLE','SS_DOUBLE','SS_DOUBLE'}),'MsgIdNumFormat',1,'MsgComment',{{''}}),'Version',1.2,'general',struct('isFromLib',0)),'OFF',[]}},'GroupId',{{struct('Group',{{'RTICAN'}},'No',1,'Behavior',{{'NAMECHANGE'}},'BlockType',{{'SINK'}},'NameChangeFlag',0),'OFF',[]}},'SFcnRTICANMessage',{{struct('MsgType','RX','SFcnPortType','Scalar','MsgName','aiBox_Front_PDO2','MsgIdFormat','STD','MsgId',641,'MsgLength',8,'NumSignals',4,'SampleTime',-1,'Signal',struct('SgnName',{'Raw_Steering_Wheel_Signal','Raw_Throttle_Pedal_2','Raw_Throttle_Pedal_1','Raw_Brake_Signal'},'SgnStartBit',{0,16,32,48},'SgnLength',{16,16,16,16},'SgnType',{'standard','standard','standard','standard'},'ModeValue',{-1,-1,-1,-1},'DataType',{['unsigned int'],['unsigned int'],['unsigned int'],['unsigned int']},'ByteLayout',{['motorola back.'],['motorola back.'],['motorola back.'],['motorola back.']},'Factor',{1,1,1,1},'Offset',{0,0,0,0},'SLDataType',{'SS_DOUBLE','SS_DOUBLE','SS_DOUBLE','SS_DOUBLE'}),'StatusSelected','yes','TimeSelected','yes','DeltaTimeSelected','yes','BytePortSelected','no','MessageLengthSelected','no','TriggerPort',struct('Selected','no','TriggerType',0),'UserCoding',struct('Selected','no','InterfaceFile','UserDecodingFile','FcnName','UserDecodeFcn','InportSelected','no','InportWidth',1,'OutportSelected','no','OutportWidth',1),'EnablePortSelected','no','UseRXService','no','BoardType','DS1','BoardNo',1,'ControllerNo',1),'OFF',[]}},'TLCFileName',{{'rtican_rx_message','OFF',[]}})  RTISFcnParameters=struct('SFcnRTICANMessage','struct','TLCFileName','char')  RTIBlockParaDefault=struct('BoardTypeNo',4302,'BoardNo',1,'ChannelNo',1,'Parameters',struct('DataFileSupport',struct('DataFileSelectedMaster',0,'DataFileSelectedLocal',0,'DataFileName','','DataFileDate','','SelectedFile',['<no file selected>']),'Options',struct('StatusSelected',1,'TimeSelected',1,'DeltaTimeSelected',1,'BytePortSelected',0,'MessageLengthSelected',0,'TriggerPort',struct('Selected',0,'TriggerType','rising'),'UserCoding',struct('Selected',0,'InterfaceFile','UserDecodingFile','FcnName','UserDecodeFcn','InportSelected',0,'InportWidth',1,'OutportSelected',0,'OutportWidth',1),'EnablePortSelected',0,'SignalOnPortnameSelected',1,'UseRXService',0),'Message',struct('MsgOnBlocknameSelected',0,'MsgName',['RX Message'],'MsgIdFormat',0,'MsgId',100,'MsgLength',8,'NumSignals',1,'SampleTime',-1,'Signal',struct('SgnName',['RX signal'],'SgnStartBit',0,'SgnLength',8,'SgnType',0,'ModeValue',-1,'DataType',0,'SLDataType','SS_DOUBLE','ByteLayout',0,'Factor',1,'Offset',0,'Min',0,'Max',255,'SgnComment',{{}},'SgnUnit',''),'MsgIdNumFormat',0,'MsgComment',{{''}}),'Version',1.2,'general',struct('isFromLib',1)),'GroupId',struct('Group',{{'RTICAN'}},'No',1,'Behavior',{{'NAMECHANGE'}},'BlockType',{{'SINK'}},'NameChangeFlag',0),'SFcnRTICANMessage',struct('MsgType','RX','MsgName',['RX Message'],'MsgIdFormat','STD','MsgId',100,'MsgLength',8,'NumSignals',1,'SampleTime',-1,'Signal',struct('SgnName',['RX signal'],'SgnStartBit',0,'SgnLength',8,'SgnType','standard','ModeValue',-1,'DataType',['unsigned int'],'ByteLayout',['little endian'],'SLDataType','SS_DOUBLE','Factor',1,'Offset',0),'StatusSelected','yes','TimeSelected','yes','DeltaTimeSelected','yes','BytePortSelected','no','MessageLengthSelected','no','EnablePortSelected','no','UserCoding',struct('Selected','no','InterfaceFile','UserDecodingFile','FcnName','UserDecodeFcn','InportSelected','no','InportWidth',1,'OutportSelected','no','OutportWidth',1),'TriggerPort',struct('Selected','no','TriggerType','rising'),'UseRXService','no','BoardType','DS4302','BoardNo',1,'ControllerNo',1,'SFcnPortType','Scalar'),'TLCFileName','rtican_rx_message')
      settings: AttributesFormatString=Group Id: RTICAN1\n
  Raw_SWS : Outport
  Raw_TP2 : Outport  Port=2
  Raw_TP1 : Outport  Port=3
  "Raw_BS " : Outport  Port=4
  RX_aiFr_PDO2_Status : Outport  Port=5
  RX_aiFr_PDO2_Time : Outport  Port=6
  RX_aiFr_PDO2_DeltaTime : Outport  Port=7
  RX_Int_aiBox_Front_PDO2 : Outport  Port=8
  wires:
  aiBox_Front_PDO2/1 -> Raw_SWS/1  "Raw_Steering_Wheel_Signal"
  aiBox_Front_PDO2/2 -> Raw_TP2/1  "Raw_Throttle_Pedal_2"
  aiBox_Front_PDO2/3 -> Raw_TP1/1  "Raw_Throttle_Pedal_1"
  aiBox_Front_PDO2/4 -> "Raw_BS "/1  "Raw_Brake_Signal"
  aiBox_Front_PDO2/5 -> RX_aiFr_PDO2_Status/1
  aiBox_Front_PDO2/6 -> RX_aiFr_PDO2_Time/1
  aiBox_Front_PDO2/7 -> RX_aiFr_PDO2_DeltaTime/1
  Switch/1 -> Memory/1, RX_Int_aiBox_Front_PDO2/1
  Memory/1 -> Switch/2
  Constant1/1 -> Switch/3
  Constant/1 -> Switch/1

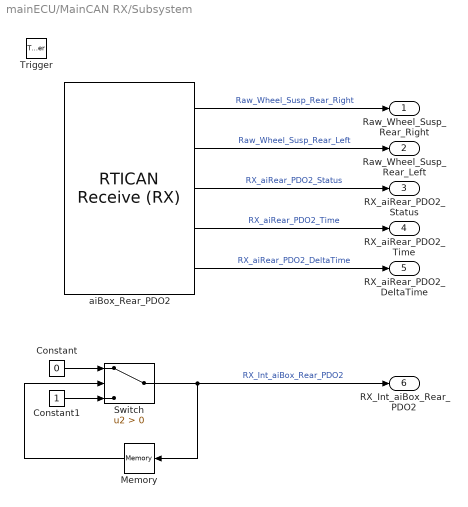
== system mainECU/MainCAN RX/Subsystem ==
  Trigger : TriggerPort  TriggerType=function-call  PortDimensions=1
  Constant : Constant  Value=0
  Constant1 : Constant
  Memory : Memory  InheritSampleTime=on
  Switch : Switch  Criteria=u2 > Threshold
  aiBox_Rear_PDO2 : rtican/RTICAN Receive (RX)   Reserved1=[]  Reserved2=[]  Reserved3=[]  Reserved4=[]  SfcnMessage=[]  Msg_Struct=[]  BoardTypeNo=[]  BoardNo=[]  ChannelNo=[]  Parameters=[]  DialogFcn=[]  UnitName=[]  Revision=[]  UnitValues=[]  DSProperties=struct('RTI',struct('Version',uint32(5),'BlockType',struct('isSLSource',uint8(1),'isSLSink',uint8(1),'isHWSource',uint8(0),'isHWSink',uint8(0),'isSetup',uint8(0),'isInline',uint8(1),'isNonInline',uint8(0),'isInterrupt',uint8(0),'isChannelwise',uint8(0)),'IOBoardType','RTICAN','UnitType','MESSAGE','Identifier','RX','DialogType','MSVC','BlockSet','RTICAN','SlaveProcessor','CAN'))  RTIBlockInterface=struct('OutputPortsWidth',int32([1 1 1 1 1]),'OutputPortsActive',[1 1 1 1 1],'OutputPortsName',{{'Raw_Wheel_Susp_Rear_Right','Raw_Wheel_Susp_Rear_Left',['RX status'],['RX time'],['RX delta time']}},'OutputPortsDataType',{{'SS_DOUBLE','SS_DOUBLE','SS_DOUBLE','SS_DOUBLE','SS_DOUBLE'}},'OutputPortsLabel',{{'Raw_Wheel_Susp_Rear_Right','Raw_Wheel_Susp_Rear_Left','','',''}},'OutputPortsLabelMode','ON','InputPortsWidth',int32(0),'InputPortsActive',0,'DialogFcn','rtican_message_interface_gui','BlockDisplay',{{'','center'}},'IconTransparency','on','ParameterTunableNames',{{}},'InitLevel',3,'BlockName',struct('Token',{{'aiBox_Rear_PDO2'}}),'SampleTime',{{-1}},'TriggerPort',{{'none'}},'EnablePort',{{'none'}})  RTIBlockParameters=struct('BoardTypeNo',{{1,'OFF',[]}},'BoardNo',{{1,'ON',[1 16]}},'ChannelNo',{{1,'ON',[1 2]}},'Parameters',{{struct('DataFileSupport',struct('DataFileSelectedMaster',1,'DataFileSelectedLocal',1,'DataFileName',['c:\users\luis\documents\tuc racing\mainecu\database\main_0_2.dbc|'],'DataFileDate',{{{['07-ene.-2017 20:06:27']}}},'SelectedFile','database\main_0_2.dbc'),'Options',struct('StatusSelected',1,'TimeSelected',1,'DeltaTimeSelected',1,'BytePortSelected',0,'MessageLengthSelected',0,'TriggerPort',struct('Selected',0,'TriggerType',0),'UserCoding',struct('Selected',0,'InterfaceFile','UserDecodingFile','FcnName','UserDecodeFcn','InportSelected',0,'InportWidth',1,'OutportSelected',0,'OutportWidth',1),'EnablePortSelected',0,'SignalOnPortnameSelected',1,'UseRXService',0),'Message',struct('MsgOnBlocknameSelected',1,'MsgName','aiBox_Rear_PDO2','MsgIdFormat',0,'MsgId',644,'MsgLength',8,'NumSignals',2,'SampleTime',-1,'Signal',struct('SgnName',{'Raw_Wheel_Susp_Rear_Right','Raw_Wheel_Susp_Rear_Left'},'SgnStartBit',{32,48},'SgnLength',{16,16},'SgnType',{0,0},'ModeValue',{-1,-1},'DataType',{0,0},'ByteLayout',{2,2},'Factor',{1,1},'Offset',{0,0},'SgnComment',{{''},{''}},'SgnUnit',{'',''},'Min',{0,0},'Max',{0,0},'SLDataType',{'SS_DOUBLE','SS_DOUBLE'}),'MsgIdNumFormat',0,'MsgComment',{{''}}),'Version',1.2,'general',struct('isFromLib',0)),'OFF',[]}},'GroupId',{{struct('Group',{{'RTICAN'}},'No',1,'Behavior',{{'NAMECHANGE'}},'BlockType',{{'SINK'}},'NameChangeFlag',0),'OFF',[]}},'SFcnRTICANMessage',{{struct('MsgType','RX','SFcnPortType','Scalar','MsgName','aiBox_Rear_PDO2','MsgIdFormat','STD','MsgId',644,'MsgLength',8,'NumSignals',2,'SampleTime',-1,'Signal',struct('SgnName',{'Raw_Wheel_Susp_Rear_Right','Raw_Wheel_Susp_Rear_Left'},'SgnStartBit',{32,48},'SgnLength',{16,16},'SgnType',{'standard','standard'},'ModeValue',{-1,-1},'DataType',{['unsigned int'],['unsigned int']},'ByteLayout',{['motorola back.'],['motorola back.']},'Factor',{1,1},'Offset',{0,0},'SLDataType',{'SS_DOUBLE','SS_DOUBLE'}),'StatusSelected','yes','TimeSelected','yes','DeltaTimeSelected','yes','BytePortSelected','no','MessageLengthSelected','no','TriggerPort',struct('Selected','no','TriggerType',0),'UserCoding',struct('Selected','no','InterfaceFile','UserDecodingFile','FcnName','UserDecodeFcn','InportSelected','no','InportWidth',1,'OutportSelected','no','OutportWidth',1),'EnablePortSelected','no','UseRXService','no','BoardType','DS1','BoardNo',1,'ControllerNo',1),'OFF',[]}},'TLCFileName',{{'rtican_rx_message','OFF',[]}})  RTISFcnParameters=struct('SFcnRTICANMessage','struct','TLCFileName','char')  RTIBlockParaDefault=struct('BoardTypeNo',4302,'BoardNo',1,'ChannelNo',1,'Parameters',struct('DataFileSupport',struct('DataFileSelectedMaster',0,'DataFileSelectedLocal',0,'DataFileName','','DataFileDate','','SelectedFile',['<no file selected>']),'Options',struct('StatusSelected',1,'TimeSelected',1,'DeltaTimeSelected',1,'BytePortSelected',0,'MessageLengthSelected',0,'TriggerPort',struct('Selected',0,'TriggerType','rising'),'UserCoding',struct('Selected',0,'InterfaceFile','UserDecodingFile','FcnName','UserDecodeFcn','InportSelected',0,'InportWidth',1,'OutportSelected',0,'OutportWidth',1),'EnablePortSelected',0,'SignalOnPortnameSelected',1,'UseRXService',0),'Message',struct('MsgOnBlocknameSelected',0,'MsgName',['RX Message'],'MsgIdFormat',0,'MsgId',100,'MsgLength',8,'NumSignals',1,'SampleTime',-1,'Signal',struct('SgnName',['RX signal'],'SgnStartBit',0,'SgnLength',8,'SgnType',0,'ModeValue',-1,'DataType',0,'SLDataType','SS_DOUBLE','ByteLayout',0,'Factor',1,'Offset',0,'Min',0,'Max',255,'SgnComment',{{}},'SgnUnit',''),'MsgIdNumFormat',0,'MsgComment',{{''}}),'Version',1.2,'general',struct('isFromLib',1)),'GroupId',struct('Group',{{'RTICAN'}},'No',1,'Behavior',{{'NAMECHANGE'}},'BlockType',{{'SINK'}},'NameChangeFlag',0),'SFcnRTICANMessage',struct('MsgType','RX','MsgName',['RX Message'],'MsgIdFormat','STD','MsgId',100,'MsgLength',8,'NumSignals',1,'SampleTime',-1,'Signal',struct('SgnName',['RX signal'],'SgnStartBit',0,'SgnLength',8,'SgnType','standard','ModeValue',-1,'DataType',['unsigned int'],'ByteLayout',['little endian'],'SLDataType','SS_DOUBLE','Factor',1,'Offset',0),'StatusSelected','yes','TimeSelected','yes','DeltaTimeSelected','yes','BytePortSelected','no','MessageLengthSelected','no','EnablePortSelected','no','UserCoding',struct('Selected','no','InterfaceFile','UserDecodingFile','FcnName','UserDecodeFcn','InportSelected','no','InportWidth',1,'OutportSelected','no','OutportWidth',1),'TriggerPort',struct('Selected','no','TriggerType','rising'),'UseRXService','no','BoardType','DS4302','BoardNo',1,'ControllerNo',1,'SFcnPortType','Scalar'),'TLCFileName','rtican_rx_message')
      settings: AttributesFormatString=Group Id: RTICAN1\n
  Raw_Wheel_Susp_Rear_Right : Outport
  Raw_Wheel_Susp_Rear_Left : Outport  Port=2
  RX_aiRear_PDO2_Status : Outport  Port=3
  RX_aiRear_PDO2_Time : Outport  Port=4
  RX_aiRear_PDO2_DeltaTime : Outport  Port=5
  RX_Int_aiBox_Rear_PDO2 : Outport  Port=6
  wires:
  aiBox_Rear_PDO2/1 -> Raw_Wheel_Susp_Rear_Right/1  "Raw_Wheel_Susp_Rear_Right"
  aiBox_Rear_PDO2/5 -> RX_aiRear_PDO2_DeltaTime/1  "RX_aiRear_PDO2_DeltaTime"
  aiBox_Rear_PDO2/3 -> RX_aiRear_PDO2_Status/1  "RX_aiRear_PDO2_Status"
  aiBox_Rear_PDO2/2 -> Raw_Wheel_Susp_Rear_Left/1  "Raw_Wheel_Susp_Rear_Left"
  aiBox_Rear_PDO2/4 -> RX_aiRear_PDO2_Time/1  "RX_aiRear_PDO2_Time"
  Switch/1 -> Memory/1, RX_Int_aiBox_Rear_PDO2/1  "RX_Int_aiBox_Rear_PDO2"
  Memory/1 -> Switch/2
  Constant1/1 -> Switch/3
  Constant/1 -> Switch/1

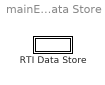
== system mainECU/RTI Data/RTI Data Store ==
  RTI Data Store : Subsystem  mask(RTI_DATA_STORE){}
      mask help:
      | RTI Data Store Block. This block is used by RTI to store internal model dependent data. Deleting this block will result in data loss.
      |
      | NEVER DELETE, COPY, OR MODIFY THIS BLOCK!
      mask Help:
      | RTI Data Store Block. This block is used by RTI to store internal model dependent data. Deleting this block will result in data loss.
      | 
      | NEVER DELETE, COPY, OR MODIFY THIS BLOCK!
      mask Display: text(0.5, 0.5, ' ', 'HorizontalAlignment', 'center');
